simulink model "simud"  (R2021a)
settings: Solver=VariableStepAuto  StartTime=0.0  StopTime=5  RelTol=1e-3
values from neighbouring files (symbols this model uses):
  Gm = Gm1    [desarrollod.m]
  K0 = -polyval(den,s)*s/polyval(num,s)    [desarrollod.m]
  K1 = -polyval(den,s)*s/polyval(num,s)    [desarrollod.m]
  Ki1 = zero*Kp1    [desarrollod.m]
  Ki2 = zero*Kp2    (= 0.0984)    [desarrollod.m]
  Kp1 = -(s*polyval(den,s))/polyval(num,s)/(s+zero)    [desarrollod.m]
  Kp2 = 0.0656    [desarrollod.m]
settings Model: Creator=pierr  LastModifiedBy=pierr

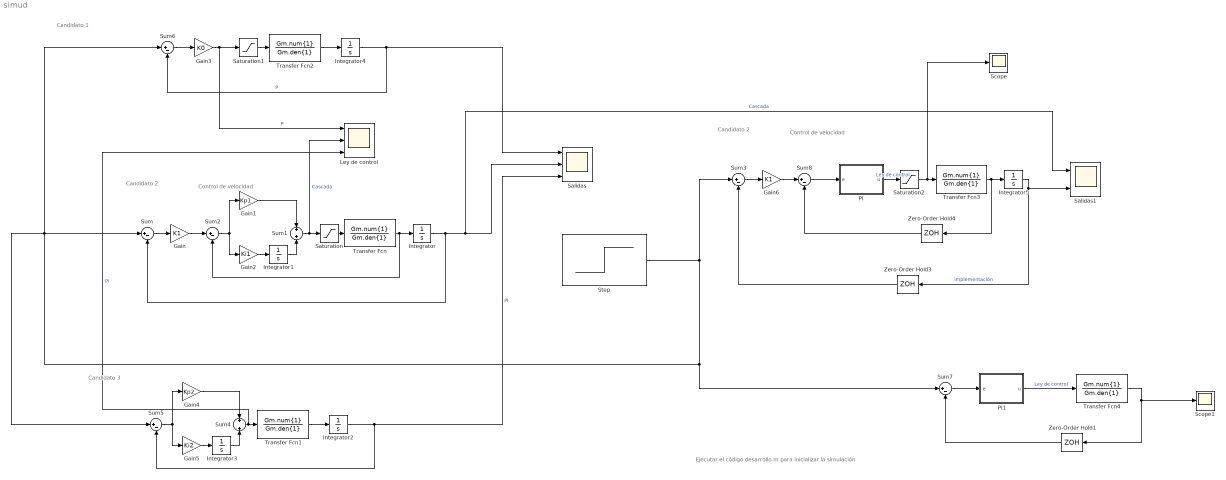
== system simud ==
  note: Ejecutar el código desarrollo.m para inicializar la simulación
  note: Candidato 3
  note: Candidato 2
  note: Candidato 1
  note: Control de velocidad
  note: Candidato 2
  note: Control de velocidad
  Gain : Gain  Gain=K1
  Gain1 : Gain  Gain=Kp1
  Gain2 : Gain  Gain=Ki1
  Gain3 : Gain  Gain=K0
  Gain4 : Gain  Gain=Kp2
  Gain5 : Gain  Gain=Ki2
  Gain6 : Gain  Gain=K1
  Integrator{,1..5} (6 alike) : Integrator
  Ley de control : Scope  NumInputPorts=3
  PI : MATLAB Function  TreatAsAtomicUnit=on
  PI1 : MATLAB Function  TreatAsAtomicUnit=on
  Salidas : Scope  NumInputPorts=3
  Salidas1 : Scope  NumInputPorts=2
  Saturation : Saturate  UpperLimit=4.8  LowerLimit=-4.8
  Saturation1 : Saturate  UpperLimit=4.8  LowerLimit=-4.8
  Saturation2 : Saturate  UpperLimit=4.8  LowerLimit=-4.8
  Scope : Scope
  Scope1 : Scope
  Step : Step  Time=0  After=-205  SampleTime=0.006
  Sum{,2..3,5..8} (7 alike) : Sum  Inputs=|+-
  Sum1 : Sum  Inputs=+||+
  Sum4 : Sum  Inputs=+||+
  Transfer Fcn{,1..4} (5 alike) : TransferFcn  Numerator=Gm.num{1}  Denominator=Gm.den{1}
  Zero-Order Hold1 : ZeroOrderHold  SampleTime=0.006
  Zero-Order Hold3 : ZeroOrderHold  SampleTime=0.006
  Zero-Order Hold4 : ZeroOrderHold  SampleTime=0.006
  wires:
  Sum/1 -> Gain/1
  Integrator/1 -> Sum/2, Salidas1/1, Salidas/2  "Cascada"
  Gain2/1 -> Integrator1/1
  Sum1/1 -> Saturation/1, Ley de control/2  "Cascada"
  Integrator1/1 -> Sum1/2
  Gain1/1 -> Sum1/1
  Gain/1 -> Sum2/1
  Sum2/1 -> Gain1/1, Gain2/1
  Sum4/1 -> Ley de control/3, Transfer Fcn1/1  "PI"
  Gain4/1 -> Sum4/1
  Sum5/1 -> Gain4/1, Gain5/1
  Integrator3/1 -> Sum4/2
  Transfer Fcn1/1 -> Integrator2/1
  Gain5/1 -> Integrator3/1
  Integrator2/1 -> Salidas/3, Sum5/2  "PI"
  Integrator4/1 -> Salidas/1, Sum6/2  "P"
  Transfer Fcn2/1 -> Integrator4/1
  Sum6/1 -> Gain3/1
  Gain3/1 -> Saturation1/1, Ley de control/1  "P"
  Saturation/1 -> Transfer Fcn/1
  Saturation1/1 -> Transfer Fcn2/1
  Transfer Fcn/1 -> Sum2/2, Integrator/1
  Zero-Order Hold3/1 -> Sum3/2
  Zero-Order Hold4/1 -> Sum8/2
  Saturation2/1 -> Scope/1, Transfer Fcn3/1
  Step/1 -> Sum7/1, Sum6/1, Sum/1, Sum5/1, Sum3/1
  Gain6/1 -> Sum8/1
  Transfer Fcn3/1 -> Zero-Order Hold4/1, Integrator5/1
  Integrator5/1 -> Salidas1/2, Zero-Order Hold3/1  "implementación"
  Sum3/1 -> Gain6/1
  Sum8/1 -> PI/1(e)
  PI/1(u) -> Saturation2/1  "Ley de control"
  Sum7/1 -> PI1/1(e)
  PI1/1(u) -> Transfer Fcn4/1  "Ley de control"
  Zero-Order Hold1/1 -> Sum7/2
  Transfer Fcn4/1 -> Scope1/1, Zero-Order Hold1/1

== matlab function simud/PI ==
  data: e input; u output
function u = fcn(e)

persistent u_1
persistent e_1
if isempty(u_1)
    u_1=0;
    e_1=0;
end
Ts=0.006;
Kp=0.020056241439231;
Ki=0.441237311663075;
u=u_1+(2*Kp+Ki*Ts)/2*e+(Ki*Ts-2*Kp)/2*e_1;
e_1=e;
u_1=u;

== matlab function simud/PI1 ==
  data: e input; u output
function u = fcn(e)

persistent u_1
persistent e_1
if isempty(u_1)
    u_1=0;
    e_1=0;
end
Ts=0.006;
Kp=0.020056241439231;
Ki=0.441237311663075;
u=u_1+(2*Kp+Ki*Ts)/2*e+(Ki*Ts-2*Kp)/2*e_1;
e_1=e;
u_1=u;
